simulink model "Simulink_Controller"  (R2022b)
settings: Solver=FixedStepAuto  StartTime=0.0  StopTime=25  FixedStep=0.001  RelTol=1e-3
undefined symbols (not defined in the file or in its folder): Standard_Devices, UDP_Protocol
libraries: sldrtlib x4, simulink x1, slpidlib x1
settings Model: Creator=User  LastModifiedBy=User

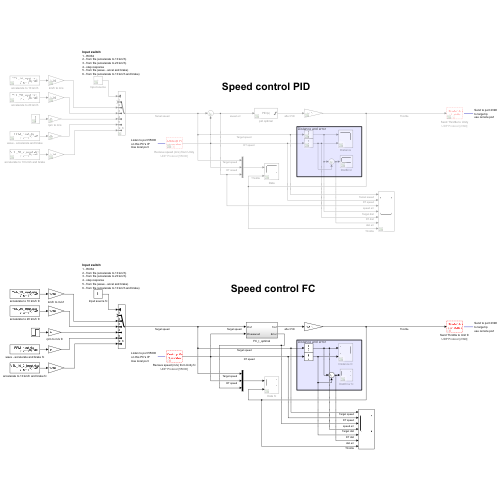
[thumbnail: Simulink's stored preview of the top-level diagram]
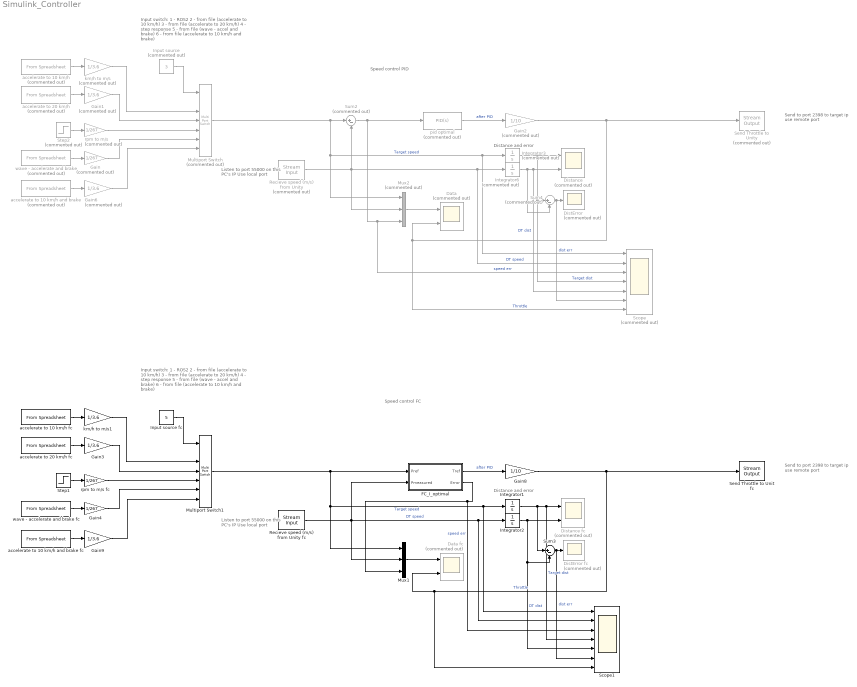
== system Simulink_Controller ==
  note: Speed control PID
  note: Input switch:
      | 1 - ROS2
      | 2 - from file (accelerate to 10 km/h)
      | 3 - from file (accelerate to 20 km/h)
      | 4 - step response
      | 5 - from file (wave - accel and brake)
      | 6 - from file (accelerate to 10 km/h and brake)
  note: Speed control FC
  note: Input switch:
      | 1 - ROS2
      | 2 - from file (accelerate to 10 km/h)
      | 3 - from file (accelerate to 20 km/h)
      | 4 - step response
      | 5 - from file (wave - accel and brake)
      | 6 - from file (accelerate to 10 km/h and brake)
  note: Listen to port 55000
      | on this PC's IP
      | Use local port
  note: Send to port 2398
      | to target ip
      | use remote port
  note: Distance and error
  note: Distance and error
  note: Listen to port 55000
      | on this PC's IP
      | Use local port
  note: Send to port 2398
      | to target ip
      | use remote port
  Data : Scope  Commented=on  NumInputPorts=2
  Data fc : Scope  Commented=on  NumInputPorts=2
  DistError : Scope  Commented=on
  DistError fc : Scope  Commented=on
  Distance : Scope  Commented=on  NumInputPorts=2
  Distance fc : Scope  Commented=on  NumInputPorts=2
  FC_I_optimal : Subsystem
  Gain : Gain  Commented=on  Gain=1/267
  Gain1 : Gain  Commented=on  Gain=1/3.6
  Gain2 : Gain  Commented=on  Gain=1/10
  Gain3 : Gain  Gain=1/3.6
  Gain4 : Gain  Gain=1/267
  Gain6 : Gain  Commented=on  Gain=1/3.6
  Gain8 : Gain  Gain=1/10
  Gain9 : Gain  Gain=1/3.6
  Input source : Constant  Commented=on  Value=3
  Input source fc : Constant  Value=5
  Integrator1 : Integrator
  Integrator2 : Integrator
  Integrator3 : Integrator  Commented=on
  Integrator6 : Integrator  Commented=on
  Multiport Switch : MultiPortSwitch  Commented=on  Inputs=6  SaturateOnIntegerOverflow=off  InputSameDT=off
  Multiport Switch1 : MultiPortSwitch  Inputs=6  SaturateOnIntegerOverflow=off  InputSameDT=off
  Mux1 : Mux  Inputs=3
  Mux2 : Mux  Commented=on  Inputs=3
  Recieve speed (m/s) from Unity : sldrtlib/Stream Input  Commented=on  SampleTime=0.005  MaxMissedTicks=100  ShowMissedTicks=off  YieldWhenWaiting=on  DrvName=Standard_Devices/UDP_Protocol  DrvAddress=55000  DrvOptions=[0 55001 0 0 0 0 0 0 0 0 0 0 0 0 0 0 0 0 0 0 0 0 0 0 0 0 0 0 0 0 0 0 0 0 0 0 0 0 0 0 0 0 0 0 0 0 0 0 0 0 0 0 0 0 0 0 0 0 0 0 0 0 0 0 0 0 0 0 0 0 0 0 0 0 0 0 0 0 0 0 0 0 0 0 0 0 0 0 0 0 0 0 0 0 0 0 0 0 0 0 0 0 0 0 0 0 0 0 0 0 0 0 0 0 0 0 0 0 0 0 0 0 0 0 0 0 0 0 0 0 0 0 0 0 0 0 0 0 0 0 0 0 0 0 0 0 0 0 0 0 0 0 0 0 0 0 0 0 0 0 0 0 0 0 0 0 0 0 0 0 0 0 0 0 0 0 0 0 0 0 0 0 0 0 0 0 0 0 0 0 0 0 0 0 0 0 0 0 0 0 0 0 0 0 0 0 0 0 0 0 0 0 0 0 0 0 0 0 0 0 0 0 0 0 0 0 0 0 0 0 0 0 0 0 0 0 0 0 0 0 0 0 0 0 0 0 0 0 0 0 0 0 0 0 0 0]  DataTypes='double'  FormatString='%f'  Terminator={'\r', '\n'}  ShowReady=off  ShowError=off
      settings: AttributesFormatString=UDP Protocol [55000]
  Recieve speed (m/s) from Unity fc : sldrtlib/Stream Input  SampleTime=0.005  MaxMissedTicks=100  ShowMissedTicks=off  YieldWhenWaiting=on  DrvName=Standard_Devices/UDP_Protocol  DrvAddress=55000  DrvOptions=[0 55001 0 0 0 0 0 0 0 0 0 0 0 0 0 0 0 0 0 0 0 0 0 0 0 0 0 0 0 0 0 0 0 0 0 0 0 0 0 0 0 0 0 0 0 0 0 0 0 0 0 0 0 0 0 0 0 0 0 0 0 0 0 0 0 0 0 0 0 0 0 0 0 0 0 0 0 0 0 0 0 0 0 0 0 0 0 0 0 0 0 0 0 0 0 0 0 0 0 0 0 0 0 0 0 0 0 0 0 0 0 0 0 0 0 0 0 0 0 0 0 0 0 0 0 0 0 0 0 0 0 0 0 0 0 0 0 0 0 0 0 0 0 0 0 0 0 0 0 0 0 0 0 0 0 0 0 0 0 0 0 0 0 0 0 0 0 0 0 0 0 0 0 0 0 0 0 0 0 0 0 0 0 0 0 0 0 0 0 0 0 0 0 0 0 0 0 0 0 0 0 0 0 0 0 0 0 0 0 0 0 0 0 0 0 0 0 0 0 0 0 0 0 0 0 0 0 0 0 0 0 0 0 0 0 0 0 0 0 0 0 0 0 0 0 0 0 0 0 0 0 0 0 0 0 0]  DataTypes='double'  FormatString='%f'  Terminator={'\r', '\n'}  ShowReady=off  ShowError=off
      settings: AttributesFormatString=UDP Protocol [55000]
  Scope : Scope  Commented=on  NumInputPorts=7
  Scope1 : Scope  NumInputPorts=7
  Send Throttle to Unit fc : sldrtlib/Stream Output  SampleTime=0.005  MaxMissedTicks=100  ShowMissedTicks=off  YieldWhenWaiting=on  DrvName=Standard_Devices/UDP_Protocol  DrvAddress=2399  DrvOptions=[0 2398 49 50 55 46 48 46 48 46 49 0 0 0 0 0 0 0 0 0 0 0 0 0 0 0 0 0 0 0 0 0 0 0 0 0 0 0 0 0 0 0 0 0 0 0 0 0 0 0 0 0 0 0 0 0 0 0 0 0 0 0 0 0 0 0 0 0 0 0 0 0 0 0 0 0 0 0 0 0 0 0 0 0 0 0 0 0 0 0 0 0 0 0 0 0 0 0 0 0 0 0 0 0 0 0 0 0 0 0 0 0 0 0 0 0 0 0 0 0 0 0 0 0 0 0 0 0 0 0 0 0 0 0 0 0 0 0 0 0 0 0 0 0 0 0 0 0 0 0 0 0 0 0 0 0 0 0 0 0 0 0 0 0 0 0 0 0 0 0 0 0 0 0 0 0 0 0 0 0 0 0 0 0 0 0 0 0 0 0 0 0 0 0 0 0 0 0 0 0 0 0 0 0 0 0 0 0 0 0 0 0 0 0 0 0 0 0 0 0 0 0 0 0 0 0 0 0 0 0 0 0 0 0 0 0 0 0 0 0 0 0 0 0 0 0 0 0 0 0 0 0 0 0 0 0]  PortSizes=1  FormatString='%f'  ShowReady=off  ShowError=off  InitialValue='2'  FinalValue=[]
      settings: AttributesFormatString=UDP Protocol [2399]
  Send Throttle to Unity : sldrtlib/Stream Output  Commented=on  SampleTime=0.005  MaxMissedTicks=100  ShowMissedTicks=off  YieldWhenWaiting=on  DrvName=Standard_Devices/UDP_Protocol  DrvAddress=2399  DrvOptions=[0 2398 49 50 55 46 48 46 48 46 49 0 0 0 0 0 0 0 0 0 0 0 0 0 0 0 0 0 0 0 0 0 0 0 0 0 0 0 0 0 0 0 0 0 0 0 0 0 0 0 0 0 0 0 0 0 0 0 0 0 0 0 0 0 0 0 0 0 0 0 0 0 0 0 0 0 0 0 0 0 0 0 0 0 0 0 0 0 0 0 0 0 0 0 0 0 0 0 0 0 0 0 0 0 0 0 0 0 0 0 0 0 0 0 0 0 0 0 0 0 0 0 0 0 0 0 0 0 0 0 0 0 0 0 0 0 0 0 0 0 0 0 0 0 0 0 0 0 0 0 0 0 0 0 0 0 0 0 0 0 0 0 0 0 0 0 0 0 0 0 0 0 0 0 0 0 0 0 0 0 0 0 0 0 0 0 0 0 0 0 0 0 0 0 0 0 0 0 0 0 0 0 0 0 0 0 0 0 0 0 0 0 0 0 0 0 0 0 0 0 0 0 0 0 0 0 0 0 0 0 0 0 0 0 0 0 0 0 0 0 0 0 0 0 0 0 0 0 0 0 0 0 0 0 0 0]  PortSizes=1  FormatString='%f'  ShowReady=off  ShowError=off  InitialValue='2'  FinalValue=[]
      settings: AttributesFormatString=UDP Protocol [2399]
  Step1 : Step  After=1100  SampleTime=0
  Step2 : Step  Commented=on  After=1100  SampleTime=0
  Sum2 : Sum  Commented=on  Inputs=|+-
  Sum3 : Sum  Inputs=|+-
  Sum4 : Sum  Commented=on  Inputs=|+-
  accelerate to 10 km/h : FromSpreadsheet  Commented=on  FileName=VEL_10_input.xlsx  SheetName=Лист1  Range=A1:B56  ExtrapolationBeforeFirstDataPoint=Hold first value  ExtrapolationAfterLastDataPoint=Hold last value
  accelerate to 10 km/h and brake : FromSpreadsheet  Commented=on  FileName=VEL_10_2_input.xlsx  SheetName=Лист1  Range=A1:B36  ExtrapolationBeforeFirstDataPoint=Hold first value  ExtrapolationAfterLastDataPoint=Hold last value
  accelerate to 10 km/h and brake fc : FromSpreadsheet  FileName=VEL_10_2_input.xlsx  SheetName=Лист1  Range=A1:B36  ExtrapolationBeforeFirstDataPoint=Hold first value  ExtrapolationAfterLastDataPoint=Hold last value
  accelerate to 10 km/h fc : FromSpreadsheet  FileName=VEL_10_input.xlsx  SheetName=Лист1  Range=A1:B56  ExtrapolationBeforeFirstDataPoint=Hold first value  ExtrapolationAfterLastDataPoint=Hold last value
  accelerate to 20 km/h : FromSpreadsheet  Commented=on  FileName=VEL_20_input.xlsx  SheetName=Лист1  Range=A1:B36  ExtrapolationBeforeFirstDataPoint=Hold first value  ExtrapolationAfterLastDataPoint=Hold last value
  accelerate to 20 km/h fc : FromSpreadsheet  FileName=VEL_20_input.xlsx  SheetName=Лист1  Range=A1:B36  ExtrapolationBeforeFirstDataPoint=Hold first value  ExtrapolationAfterLastDataPoint=Hold last value
  km/h to m/s : Gain  Commented=on  Gain=1/3.6
  km/h to m/s1 : Gain  Gain=1/3.6
  pid optimal : slpidlib/PID Controller  Commented=on  Controller=PID  Form=Parallel  TimeDomain=Continuous-time  UseExternalTs=off  SampleTime=0.1  IntegratorMethod=Forward Euler  FilterMethod=Forward Euler  ControllerParametersSource=internal  P=10  I=40  UseKiTs=off  D=0  N=0  UseFilter=on  TunerSelectOption=Transfer Function Based (PID Tuner App)  InitialConditionSource=internal  InitialConditionForIntegrator=0  InitialConditionForFilter=0  DifferentiatorICPrevScaledInput=0  ExternalReset=none  TrackingMode=off  Kt=1  LimitOutput=on  SatLimitsSource=internal  UpperSaturationLimit=10  LowerSaturationLimit=-10  LinearizeAsGain=off  AntiWindupMode=none  Kb=1  LimitIntegrator=off  UpperIntegratorSaturationLimit=inf  LowerIntegratorSaturationLimit=-inf  POutMin=[]  POutMax=[]  IOutMin=[]  IOutMax=[]  DOutMin=[]  DOutMax=[]  NOutMin=[]  NOutMax=[]  SumOutMin=[]  SumOutMax=[]  SaturationOutMin=[]  SaturationOutMax=[]  PParamMin=[]  PParamMax=[]  IParamMin=[]  IParamMax=[]  DParamMin=[]  DParamMax=[]  NParamMin=[]  NParamMax=[]  KbParamMin=[]  KbParamMax=[]  KtParamMin=[]  KtParamMax=[]  KbOutMin=[]  KbOutMax=[]  KtOutMin=[]  KtOutMax=[]  IntegratorOutMin=[]  IntegratorOutMax=[]  FilterOutMin=[]  FilterOutMax=[]  SumI1OutMin=[]  SumI1OutMax=[]  SumI2OutMin=[]  SumI2OutMax=[]  SumI3OutMin=[]  SumI3OutMax=[]  SumI4OutMin=[]  SumI4OutMax=[]  SumDOutMin=[]  SumDOutMax=[]  DifferentiatorOutMin=[]  DifferentiatorOutMax=[]  FilterDiffOutCoefMin=[]  FilterDiffOutCoefMax=[]  ReciprocalOutMin=[]  ReciprocalOutMax=[]  SumDenOutMin=[]  SumDenOutMax=[]  SumNumOutMin=[]  SumNumOutMax=[]  DivideOutMin=[]  DivideOutMax=[]  UdiffTsProdOutMin=[]  UdiffTsProdOutMax=[]  NTsProdOutMin=[]  NTsProdOutMax=[]  UintegralTsProdOutMin=[]  UintegralTsProdOutMax=[]  UngainTsProdOutMin=[]  UngainTsProdOutMax=[]  ClampingZeroOutDataTypeStr=Inherit: Inherit via back propagation  ClampingZeroOutMin=[]  ClampingZeroOutMax=[]  FilterDenConstantOutDataTypeStr=Inherit: Inherit via back propagation  FilterDenConstantOutMin=[]  FilterDenConstantOutMax=[]  PCopyOutDataTypeStr=Inherit: Inherit via back propagation  PCopyOutMin=[]  PCopyOutMax=[]  NCopyOutDataTypeStr=Inherit: Inherit via back propagation  NCopyOutMin=[]  NCopyOutMax=[]  IntegratorContinuousStateAttributes=''  IntegratorStateMustResolveToSignalObject=off  IntegratorRTWStateStorageClass=Auto  FilterContinuousStateAttributes=''  FilterStateMustResolveToSignalObject=off  FilterRTWStateStorageClass=Auto  ParallelPVariant=InternalParameters  IdealPVariant=Disabled  IVariant=InternalParameters  DVariant=InternalParameters  IntegratorVariant=Continuous  SatVariant=Enabled  AWVariant=Passthrough  PCopyVariant=Disabled  TRVariant=Disabled  FdbkBlocksVariant=Forward  IdealPFdbkVariant=Disabled  SatFdbkVariant=Disabled  DerivativeFilterVariant=ContFilter  NVariant=InternalParameters  NCopyVariant=Disabled  FilterICVariant=InternalICsFilter  IntegratorICVariant=InternalICs  ExternalResetVariant=Disabled  TRSumVariant=Passthrough  SumFdbkVariant=Disabled  SumVariant=Sum_PID  TsampFilterVariant=InternalTs  TsampNgainVariant=Passthrough  TsampIntegralVariant=Passthrough  ExternalSaturationOutDataTypeStr=Inherit: Same as second input
  rpm to m/s : Gain  Commented=on  Gain=1/267
  rpm to m/s fc : Gain  Gain=1/267
  wave - accelerate and brake : FromSpreadsheet  Commented=on  FileName=RPM_input.xlsx  SheetName=Лист1  Range=A1:B4401  ExtrapolationBeforeFirstDataPoint=Hold first value  ExtrapolationAfterLastDataPoint=Hold last value
  wave - accelerate and brake fc : FromSpreadsheet  FileName=RPM_input.xlsx  SheetName=Лист1  Range=A1:B4401  ExtrapolationBeforeFirstDataPoint=Hold first value  ExtrapolationAfterLastDataPoint=Hold last value
  wires:
  Gain3/1 -> Multiport Switch1/4
  Sum3/1 -> Scope1/6, DistError fc/1  "dist err"
  Gain8/1 -> Send Throttle to Unit fc/1, Scope1/7, Data fc/2  "Throttle"
  Gain4/1 -> Multiport Switch1/6
  Integrator2/1 -> Scope1/5, Sum3/2, Distance fc/2  "DT dist"
  Sum2/1 -> pid optimal/1, Scope/3, Mux2/3  "speed err"
  pid optimal/1 -> Gain2/1  "after PID"
  accelerate to 10 km/h fc/1 -> km/h to m/s1/1
  FC_I_optimal/1(Tref) -> Gain8/1  "after PID"
  wave - accelerate and brake fc/1 -> Gain4/1
  Integrator3/1 -> Scope/4, Sum4/1, Distance/1  "Target dist"
  Gain9/1 -> Multiport Switch1/7
  Mux1/1 -> Data fc/1
  Mux2/1 -> Data/1
  Gain6/1 -> Multiport Switch/7
  Multiport Switch1/1 -> FC_I_optimal/1(Pref), Scope1/1, Integrator1/1, Mux1/1  "Target speed"
  Gain1/1 -> Multiport Switch/4
  Input source fc/1 -> Multiport Switch1/1
  accelerate to 20 km/h/1 -> Gain1/1
  accelerate to 10 km/h/1 -> km/h to m/s/1
  Gain/1 -> Multiport Switch/6
  Integrator1/1 -> Sum3/1, Distance fc/1, Scope1/4  "Target dist"
  Recieve speed (m/s) from Unity/1 -> Scope/2, Integrator6/1, Mux2/2, Sum2/2  "DT speed"
  Gain2/1 -> Send Throttle to Unity/1, Scope/7, Data/2  "Throttle"
  km/h to m/s/1 -> Multiport Switch/3
  accelerate to 10 km/h and brake/1 -> Gain6/1
  km/h to m/s1/1 -> Multiport Switch1/3
  Sum4/1 -> Scope/6, DistError/1  "dist err"
  Input source/1 -> Multiport Switch/1
  Step2/1 -> rpm to m/s/1
  accelerate to 10 km/h and brake fc/1 -> Gain9/1
  rpm to m/s fc/1 -> Multiport Switch1/5
  wave - accelerate and brake/1 -> Gain/1
  Integrator6/1 -> Sum4/2, Scope/5, Distance/2  "DT dist"
  rpm to m/s/1 -> Multiport Switch/5
  accelerate to 20 km/h fc/1 -> Gain3/1
  Step1/1 -> rpm to m/s fc/1
  Recieve speed (m/s) from Unity fc/1 -> FC_I_optimal/2(Pmeasured), Scope1/2, Integrator2/1, Mux1/2  "DT speed"
  FC_I_optimal/2(Error) -> Scope1/3, Mux1/3  "speed err"
  Multiport Switch/1 -> Scope/1, Integrator3/1, Mux2/1, Sum2/1  "Target speed"

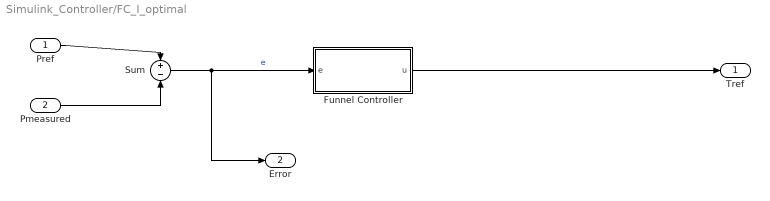
== system Simulink_Controller/FC_I_optimal ==
  Pref : Inport
  Pmeasured : Inport  Port=2
  Funnel Controller : Subsystem
  Sum : Sum  Inputs=+-
  Tref : Outport
  Error : Outport  Port=2
  wires:
  Funnel Controller/1(u) -> Tref/1
  Sum/1 -> Error/1, Funnel Controller/1(e)  "e"
  Pmeasured/1 -> Sum/2
  Pref/1 -> Sum/1

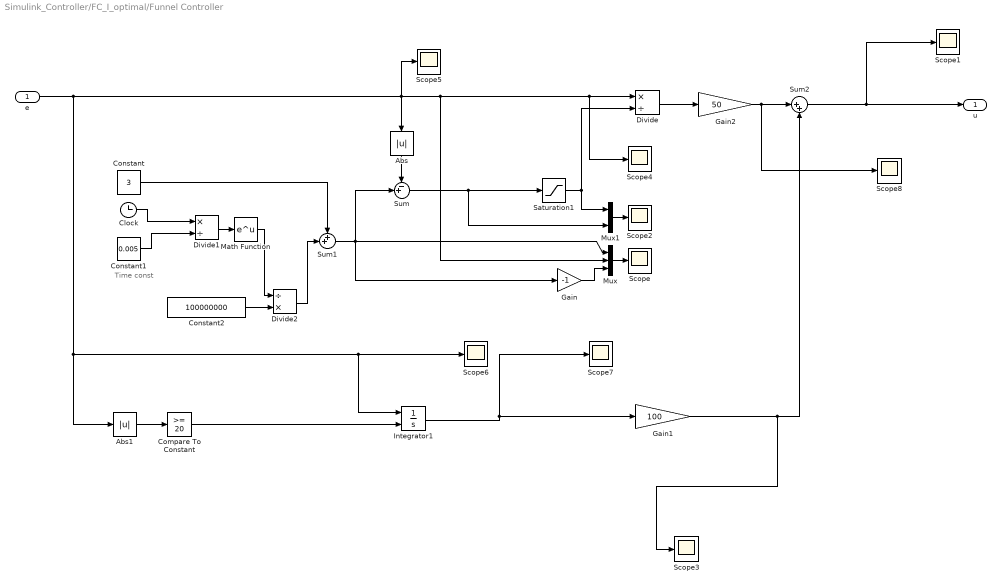
== system Simulink_Controller/FC_I_optimal/Funnel Controller ==
  note: Time const
  e : Inport
  Abs : Abs  SaturateOnIntegerOverflow=off
  Abs1 : Abs  SaturateOnIntegerOverflow=off
  Clock : Clock
  Compare To Constant : simulink/Logic and Bit Operations/Compare To Constant  relop=>=  const=20  OutDataTypeStr=boolean
  Constant : Constant  Value=3
  Constant1 : Constant  Value=0.005
  Constant2 : Constant  Value=100000000
  Divide : Product  Inputs=*/
  Divide1 : Product  Inputs=*/
  Divide2 : Product  Inputs=/*
  Gain : Gain  Gain=-1
  Gain1 : Gain  Gain=100
  Gain2 : Gain  Gain=50
  Integrator1 : Integrator  ExternalReset=rising
  Math Function : Math  SignedPower=on
  Mux : Mux  Inputs=3
  Mux1 : Mux  Inputs=2
  Saturation1 : Saturate  UpperLimit=inf  LowerLimit=2
  Scope{,1..8} (9 alike) : Scope
  Sum : Sum  Inputs=-+|
  Sum1 : Sum  Inputs=++|
  Sum2 : Sum  Inputs=|++
  u : Outport
  wires:
  Saturation1/1 -> Divide/2, Mux1/1
  Mux1/1 -> Scope2/1
  Sum/1 -> Mux1/2, Saturation1/1
  Sum1/1 -> Sum/2, Mux/1, Gain/1
  Divide2/1 -> Sum1/2
  Constant2/1 -> Divide2/2
  Math Function/1 -> Divide2/1
  Divide1/1 -> Math Function/1
  Constant1/1 -> Divide1/2
  Clock/1 -> Divide1/1
  Gain/1 -> Mux/3
  Mux/1 -> Scope/1
  Constant/1 -> Sum1/1
  Abs/1 -> Sum/1
  Divide/1 -> Gain2/1
  Sum2/1 -> Scope1/1, u/1
  e/1 -> Scope5/1, Mux/2, Divide/1, Scope4/1, Abs/1, Abs1/1, Integrator1/1, Scope6/1
  Integrator1/1 -> Scope7/1, Gain1/1
  Gain1/1 -> Scope3/1, Sum2/2
  Gain2/1 -> Scope8/1, Sum2/1
  Abs1/1 -> Compare To Constant/1
  Compare To Constant/1 -> Integrator1/2
